simulink model "Lab2_2_sim_2014b"  (R2014b)
settings: Solver=ode45  StartTime=0.0  StopTime=0.1  RelTol=1e-3
settings Model: CovSFcnEnable=on  Creator=Yash Bansod  LastModifiedBy=Yash Bansod
settings DataIOCC: SaveFormat=StructureWithTime
settings DebuggingCC: SolverPrmCheckMsg=none  FrameProcessingCompatibilityMsg=error
settings HardwareCC: ProdBitPerPointer=64  ProdLargestAtomicFloat=Float  ProdIntDivRoundTo=Zero  ProdEndianess=LittleEndian  ProdHWDeviceType=Specified
settings GRTTargetCC: GeneratePreprocessorConditionals=Use local settings

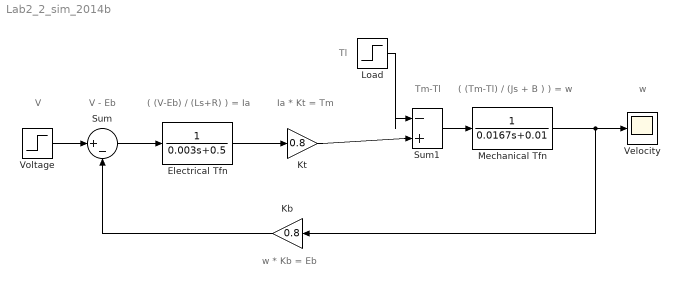
== system Lab2_2_sim_2014b ==
  note: Tm-Tl
  note: Tl
  note: V
  note: V - Eb
  note: ( (V-Eb) / (Ls+R) ) = Ia
  note: Ia * Kt = Tm
  note: ( (Tm-Tl) / (Js + B ) ) = w
  note: w
  note: w * Kb = Eb
  Electrical Tfn : TransferFcn  Denominator=[0.003 0.5]
  Kb : Gain  Gain=0.8
  Kt : Gain  Gain=0.8
  Load : Step  Time=0.015  After=100  SampleTime=0
  "Mechanical Tfn " : TransferFcn  Denominator=[0.0167 0.01]
  Sum : Sum  Inputs=|+-
  Sum1 : Sum  Inputs=|-+
  Velocity : Scope
      settings: TimeRange=auto  MaxDataPoints=5000  SaveToWorkspace=off  SaveName=ScopeData  YMin=-188.56099  YMax=270.96946  SampleInput=on  SampleTime=0.0001
  Voltage : Step  Time=0  After=220  SampleTime=0
  wires:
  Sum/1 -> Electrical Tfn/1
  Voltage/1 -> Sum/1
  Electrical Tfn/1 -> Kt/1
  "Mechanical Tfn "/1 -> Kb/1, Velocity/1
  Kb/1 -> Sum/2
  Sum1/1 -> "Mechanical Tfn "/1
  Kt/1 -> Sum1/2
  Load/1 -> Sum1/1
